simulink model "NHR9410Model96k_2020b"  (R2020b)
settings: Solver=ode45  StartTime=0.0  StopTime=1  FixedStep=0.001  MaxStep=20e-6  RelTol=1e-3
undefined symbols (not defined in the file): Ts
libraries: simulink x85, fl_lib x49, powerlib_meascontrol x27, simulink_extras x24, nesl_utility x13
(part 4 of 4)

== system NHR9410Model96k_2020b/NHR 9410 Safety Settings/Safety Ch-2/Trip signal generator (max) Sink Power/trip signal gen ==
  signal in : Inport
  Enable : EnablePort
  -1 : Constant  OutDataTypeStr=boolean
  -2 : Constant  OutDataTypeStr=boolean
  -3 : Constant  OutDataTypeStr=boolean
  -4 : Constant  Value=0  OutDataTypeStr=boolean
  -5 : Constant  Value=0  OutDataTypeStr=boolean
  -7 : Constant  Value=trip_t  OutDataTypeStr=boolean
  Add : Sum
  Compare To Constant : simulink/Logic and Bit Operations/Compare To Constant  relop=>  const=0  OutDataTypeStr=uint8
  Compare To Constant1 : simulink/Logic and Bit Operations/Compare To Constant  relop===  const=0  OutDataTypeStr=uint8
  D Latch1 : simulink_extras/Flip Flops/D Latch
      settings: SourceProductBaseCode=SL
  Data Type Conversion : DataTypeConversion  OutDataTypeStr=double
  Data Type Conversion1 : DataTypeConversion  OutDataTypeStr=double
  Gain : Gain  Gain=2
  Gain1 : Gain
  Logical Operator1 : Logic  AllPortsSameDT=off  OutDataTypeStr=boolean
  Multiport Switch : MultiPortSwitch  Inputs=2  DataPortForDefault=Additional data port
  On Delay : powerlib_meascontrol/Logic/On Delay  DelayType=On delay  delay=trip_t  ic=0  Ts=0
  Switch : Switch  Criteria=u2 > Threshold  Threshold=trip_thres
  Terminator1 : Terminator
  trip_out : Outport  VectorParamsAs1DForOutWhenUnconnected=off
  wires:
  Switch/1 -> On Delay/1, Logical Operator1/2
  On Delay/1 -> D Latch1/2
  D Latch1/1 -> Multiport Switch/2
  -4/1 -> Multiport Switch/4
  Multiport Switch/1 -> trip_out/1
  -2/1 -> Multiport Switch/3
  -3/1 -> Switch/1
  -5/1 -> Switch/3
  Logical Operator1/1 -> D Latch1/1
  D Latch1/2 -> Terminator1/1
  signal in/1 -> Switch/2
  -1/1 -> Logical Operator1/1
  -7/1 -> Compare To Constant1/1, Compare To Constant/1
  Gain1/1 -> Add/1
  Data Type Conversion/1 -> Gain1/1
  Add/1 -> Multiport Switch/1
  Gain/1 -> Add/2
  Data Type Conversion1/1 -> Gain/1
  Compare To Constant1/1 -> Data Type Conversion1/1
  Compare To Constant/1 -> Data Type Conversion/1

== system NHR9410Model96k_2020b/NHR 9410 Safety Settings/Safety Ch-2/Trip signal generator (max) Source Current/trip signal gen ==
  signal in : Inport
  Enable : EnablePort
  -1 : Constant  OutDataTypeStr=boolean
  -2 : Constant  OutDataTypeStr=boolean
  -3 : Constant  OutDataTypeStr=boolean
  -4 : Constant  Value=0  OutDataTypeStr=boolean
  -5 : Constant  Value=0  OutDataTypeStr=boolean
  -7 : Constant  Value=trip_t  OutDataTypeStr=boolean
  Add : Sum
  Compare To Constant : simulink/Logic and Bit Operations/Compare To Constant  relop=>  const=0  OutDataTypeStr=uint8
  Compare To Constant1 : simulink/Logic and Bit Operations/Compare To Constant  relop===  const=0  OutDataTypeStr=uint8
  D Latch1 : simulink_extras/Flip Flops/D Latch
      settings: SourceProductBaseCode=SL
  Data Type Conversion : DataTypeConversion  OutDataTypeStr=double
  Data Type Conversion1 : DataTypeConversion  OutDataTypeStr=double
  Gain : Gain  Gain=2
  Gain1 : Gain
  Logical Operator1 : Logic  AllPortsSameDT=off  OutDataTypeStr=boolean
  Multiport Switch : MultiPortSwitch  Inputs=2  DataPortForDefault=Additional data port
  On Delay : powerlib_meascontrol/Logic/On Delay  DelayType=On delay  delay=trip_t  ic=0  Ts=0
  Switch : Switch  Criteria=u2 > Threshold  Threshold=trip_thres
  Terminator1 : Terminator
  trip_out : Outport  VectorParamsAs1DForOutWhenUnconnected=off
  wires:
  Switch/1 -> On Delay/1, Logical Operator1/2
  On Delay/1 -> D Latch1/2
  D Latch1/1 -> Multiport Switch/2
  -4/1 -> Multiport Switch/4
  Multiport Switch/1 -> trip_out/1
  -2/1 -> Multiport Switch/3
  -3/1 -> Switch/1
  -5/1 -> Switch/3
  Logical Operator1/1 -> D Latch1/1
  D Latch1/2 -> Terminator1/1
  signal in/1 -> Switch/2
  -1/1 -> Logical Operator1/1
  -7/1 -> Compare To Constant1/1, Compare To Constant/1
  Gain1/1 -> Add/1
  Data Type Conversion/1 -> Gain1/1
  Add/1 -> Multiport Switch/1
  Gain/1 -> Add/2
  Data Type Conversion1/1 -> Gain/1
  Compare To Constant1/1 -> Data Type Conversion1/1
  Compare To Constant/1 -> Data Type Conversion/1

== system NHR9410Model96k_2020b/NHR 9410 Safety Settings/Safety Ch-2/Trip signal generator (max) Source Power/trip signal gen ==
  signal in : Inport
  Enable : EnablePort
  -1 : Constant  OutDataTypeStr=boolean
  -2 : Constant  OutDataTypeStr=boolean
  -3 : Constant  OutDataTypeStr=boolean
  -4 : Constant  Value=0  OutDataTypeStr=boolean
  -5 : Constant  Value=0  OutDataTypeStr=boolean
  -7 : Constant  Value=trip_t  OutDataTypeStr=boolean
  Add : Sum
  Compare To Constant : simulink/Logic and Bit Operations/Compare To Constant  relop=>  const=0  OutDataTypeStr=uint8
  Compare To Constant1 : simulink/Logic and Bit Operations/Compare To Constant  relop===  const=0  OutDataTypeStr=uint8
  D Latch1 : simulink_extras/Flip Flops/D Latch
      settings: SourceProductBaseCode=SL
  Data Type Conversion : DataTypeConversion  OutDataTypeStr=double
  Data Type Conversion1 : DataTypeConversion  OutDataTypeStr=double
  Gain : Gain  Gain=2
  Gain1 : Gain
  Logical Operator1 : Logic  AllPortsSameDT=off  OutDataTypeStr=boolean
  Multiport Switch : MultiPortSwitch  Inputs=2  DataPortForDefault=Additional data port
  On Delay : powerlib_meascontrol/Logic/On Delay  DelayType=On delay  delay=trip_t  ic=0  Ts=0
  Switch : Switch  Criteria=u2 > Threshold  Threshold=trip_thres
  Terminator1 : Terminator
  trip_out : Outport  VectorParamsAs1DForOutWhenUnconnected=off
  wires:
  -1/1 -> Logical Operator1/1
  signal in/1 -> Switch/2
  D Latch1/2 -> Terminator1/1
  Logical Operator1/1 -> D Latch1/1
  -5/1 -> Switch/3
  -3/1 -> Switch/1
  -2/1 -> Multiport Switch/3
  Multiport Switch/1 -> trip_out/1
  -4/1 -> Multiport Switch/4
  D Latch1/1 -> Multiport Switch/2
  On Delay/1 -> D Latch1/2
  Switch/1 -> Logical Operator1/2, On Delay/1
  -7/1 -> Compare To Constant1/1, Compare To Constant/1
  Gain1/1 -> Add/1
  Data Type Conversion/1 -> Gain1/1
  Add/1 -> Multiport Switch/1
  Gain/1 -> Add/2
  Data Type Conversion1/1 -> Gain/1
  Compare To Constant1/1 -> Data Type Conversion1/1
  Compare To Constant/1 -> Data Type Conversion/1

== system NHR9410Model96k_2020b/NHR 9410 Safety Settings/Safety Ch-2/Trip signal generator (max) Voltage/trip signal gen ==
  signal in : Inport
  Enable : EnablePort
  -1 : Constant  OutDataTypeStr=boolean
  -2 : Constant  OutDataTypeStr=boolean
  -3 : Constant  OutDataTypeStr=boolean
  -4 : Constant  Value=0  OutDataTypeStr=boolean
  -5 : Constant  Value=0  OutDataTypeStr=boolean
  -7 : Constant  Value=trip_t  OutDataTypeStr=boolean
  Add : Sum
  Compare To Constant : simulink/Logic and Bit Operations/Compare To Constant  relop=>  const=0  OutDataTypeStr=uint8
  Compare To Constant1 : simulink/Logic and Bit Operations/Compare To Constant  relop===  const=0  OutDataTypeStr=uint8
  D Latch1 : simulink_extras/Flip Flops/D Latch
      settings: SourceProductBaseCode=SL
  Data Type Conversion : DataTypeConversion  OutDataTypeStr=double
  Data Type Conversion1 : DataTypeConversion  OutDataTypeStr=double
  Gain : Gain  Gain=2
  Gain1 : Gain
  Logical Operator1 : Logic  AllPortsSameDT=off  OutDataTypeStr=boolean
  Multiport Switch : MultiPortSwitch  Inputs=2  DataPortForDefault=Additional data port
  On Delay : powerlib_meascontrol/Logic/On Delay  DelayType=On delay  delay=trip_t  ic=0  Ts=0
  Switch : Switch  Criteria=u2 > Threshold  Threshold=trip_thres
  Terminator1 : Terminator
  trip_out : Outport  VectorParamsAs1DForOutWhenUnconnected=off
  wires:
  -1/1 -> Logical Operator1/1
  signal in/1 -> Switch/2
  D Latch1/2 -> Terminator1/1
  Logical Operator1/1 -> D Latch1/1
  -5/1 -> Switch/3
  -3/1 -> Switch/1
  -2/1 -> Multiport Switch/3
  Multiport Switch/1 -> trip_out/1
  -4/1 -> Multiport Switch/4
  D Latch1/1 -> Multiport Switch/2
  On Delay/1 -> D Latch1/2
  Switch/1 -> Logical Operator1/2, On Delay/1
  -7/1 -> Compare To Constant1/1, Compare To Constant/1
  Gain1/1 -> Add/1
  Data Type Conversion/1 -> Gain1/1
  Add/1 -> Multiport Switch/1
  Gain/1 -> Add/2
  Data Type Conversion1/1 -> Gain/1
  Compare To Constant1/1 -> Data Type Conversion1/1
  Compare To Constant/1 -> Data Type Conversion/1

== system NHR9410Model96k_2020b/NHR 9410 Safety Settings/Safety Ch-2/Trip signal generator (min) Voltage/trip signal gen ==
  signal in : Inport
  Enable : EnablePort
  -1 : Constant  OutDataTypeStr=boolean
  -2 : Constant  OutDataTypeStr=boolean
  -3 : Constant  Value=0  OutDataTypeStr=boolean
  -4 : Constant  Value=0  OutDataTypeStr=boolean
  -5 : Constant  OutDataTypeStr=boolean
  -7 : Constant  Value=trip_t  OutDataTypeStr=boolean
  Add : Sum
  Compare To Constant : simulink/Logic and Bit Operations/Compare To Constant  relop=>  const=0  OutDataTypeStr=uint8
  Compare To Constant1 : simulink/Logic and Bit Operations/Compare To Constant  relop===  const=0  OutDataTypeStr=uint8
  D Latch1 : simulink_extras/Flip Flops/D Latch
      settings: SourceProductBaseCode=SL
  Data Type Conversion : DataTypeConversion  OutDataTypeStr=double
  Data Type Conversion1 : DataTypeConversion  OutDataTypeStr=double
  Gain : Gain  Gain=2
  Gain1 : Gain
  Logical Operator1 : Logic  AllPortsSameDT=off  OutDataTypeStr=boolean
  Multiport Switch : MultiPortSwitch  Inputs=2  DataPortForDefault=Additional data port
  On Delay : powerlib_meascontrol/Logic/On Delay  DelayType=On delay  delay=trip_t  ic=0  Ts=0
  Switch : Switch  Criteria=u2 > Threshold  Threshold=trip_thres
  Terminator1 : Terminator
  trip_out : Outport  VectorParamsAs1DForOutWhenUnconnected=off
  wires:
  Switch/1 -> On Delay/1, Logical Operator1/2
  On Delay/1 -> D Latch1/2
  D Latch1/1 -> Multiport Switch/2
  -4/1 -> Multiport Switch/4
  Multiport Switch/1 -> trip_out/1
  -2/1 -> Multiport Switch/3
  -3/1 -> Switch/1
  -5/1 -> Switch/3
  Logical Operator1/1 -> D Latch1/1
  D Latch1/2 -> Terminator1/1
  signal in/1 -> Switch/2
  -1/1 -> Logical Operator1/1
  -7/1 -> Compare To Constant1/1, Compare To Constant/1
  Gain1/1 -> Add/1
  Data Type Conversion/1 -> Gain1/1
  Add/1 -> Multiport Switch/1
  Gain/1 -> Add/2
  Data Type Conversion1/1 -> Gain/1
  Compare To Constant1/1 -> Data Type Conversion1/1
  Compare To Constant/1 -> Data Type Conversion/1

== system NHR9410Model96k_2020b/NHR 9410 Safety Settings/Safety Ch-2/Trip signal generator (peak) Current/trip signal gen ==
  signal in : Inport
  Enable : EnablePort
  -2 : Constant  OutDataTypeStr=boolean
  -4 : Constant  Value=0  OutDataTypeStr=boolean
  D Latch1 : simulink_extras/Flip Flops/D Latch
      settings: SourceProductBaseCode=SL
  Data Type Conversion : DataTypeConversion  OutDataTypeStr=boolean
  Switch1 : Switch  Criteria=u2 > Threshold  Threshold=trip_thres
  Terminator1 : Terminator
  trip_out : Outport  VectorParamsAs1DForOutWhenUnconnected=off
  wires:
  -4/1 -> Switch1/3
  Switch1/1 -> D Latch1/2, Data Type Conversion/1
  D Latch1/1 -> trip_out/1
  D Latch1/2 -> Terminator1/1
  -2/1 -> Switch1/1
  Data Type Conversion/1 -> D Latch1/1
  signal in/1 -> Switch1/2

== system NHR9410Model96k_2020b/NHR 9410 Safety Settings/Safety Ch-2/Trip signal generator (peak) Voltage/trip signal gen ==
  signal in : Inport
  Enable : EnablePort
  -2 : Constant  OutDataTypeStr=boolean
  -4 : Constant  Value=0  OutDataTypeStr=boolean
  D Latch1 : simulink_extras/Flip Flops/D Latch
      settings: SourceProductBaseCode=SL
  Data Type Conversion : DataTypeConversion  OutDataTypeStr=boolean
  Switch1 : Switch  Criteria=u2 > Threshold  Threshold=trip_thres
  Terminator1 : Terminator
  trip_out : Outport  VectorParamsAs1DForOutWhenUnconnected=off
  wires:
  -4/1 -> Switch1/3
  Switch1/1 -> D Latch1/2, Data Type Conversion/1
  D Latch1/1 -> trip_out/1
  D Latch1/2 -> Terminator1/1
  -2/1 -> Switch1/1
  Data Type Conversion/1 -> D Latch1/1
  signal in/1 -> Switch1/2

== system NHR9410Model96k_2020b/NHR 9410 Safety Settings/Safety Ch-3/Trip signal generator (max) Sink Current/trip signal gen ==
  signal in : Inport
  Enable : EnablePort
  -1 : Constant  OutDataTypeStr=boolean
  -2 : Constant  OutDataTypeStr=boolean
  -3 : Constant  OutDataTypeStr=boolean
  -4 : Constant  Value=0  OutDataTypeStr=boolean
  -5 : Constant  Value=0  OutDataTypeStr=boolean
  -7 : Constant  Value=trip_t  OutDataTypeStr=boolean
  Add : Sum
  Compare To Constant : simulink/Logic and Bit Operations/Compare To Constant  relop=>  const=0  OutDataTypeStr=uint8
  Compare To Constant1 : simulink/Logic and Bit Operations/Compare To Constant  relop===  const=0  OutDataTypeStr=uint8
  D Latch1 : simulink_extras/Flip Flops/D Latch
      settings: SourceProductBaseCode=SL
  Data Type Conversion : DataTypeConversion  OutDataTypeStr=double
  Data Type Conversion1 : DataTypeConversion  OutDataTypeStr=double
  Gain : Gain  Gain=2
  Gain1 : Gain
  Logical Operator1 : Logic  AllPortsSameDT=off  OutDataTypeStr=boolean
  Multiport Switch : MultiPortSwitch  Inputs=2  DataPortForDefault=Additional data port
  On Delay : powerlib_meascontrol/Logic/On Delay  DelayType=On delay  delay=trip_t  ic=0  Ts=0
  Switch : Switch  Criteria=u2 > Threshold  Threshold=trip_thres
  Terminator1 : Terminator
  trip_out : Outport  VectorParamsAs1DForOutWhenUnconnected=off
  wires:
  Switch/1 -> On Delay/1, Logical Operator1/2
  On Delay/1 -> D Latch1/2
  D Latch1/1 -> Multiport Switch/2
  -4/1 -> Multiport Switch/4
  Multiport Switch/1 -> trip_out/1
  -2/1 -> Multiport Switch/3
  -3/1 -> Switch/1
  -5/1 -> Switch/3
  Logical Operator1/1 -> D Latch1/1
  D Latch1/2 -> Terminator1/1
  signal in/1 -> Switch/2
  -1/1 -> Logical Operator1/1
  -7/1 -> Compare To Constant1/1, Compare To Constant/1
  Gain1/1 -> Add/1
  Data Type Conversion/1 -> Gain1/1
  Add/1 -> Multiport Switch/1
  Gain/1 -> Add/2
  Data Type Conversion1/1 -> Gain/1
  Compare To Constant1/1 -> Data Type Conversion1/1
  Compare To Constant/1 -> Data Type Conversion/1

== system NHR9410Model96k_2020b/NHR 9410 Safety Settings/Safety Ch-3/Trip signal generator (max) Sink Power/trip signal gen ==
  signal in : Inport
  Enable : EnablePort
  -1 : Constant  OutDataTypeStr=boolean
  -2 : Constant  OutDataTypeStr=boolean
  -3 : Constant  OutDataTypeStr=boolean
  -4 : Constant  Value=0  OutDataTypeStr=boolean
  -5 : Constant  Value=0  OutDataTypeStr=boolean
  -7 : Constant  Value=trip_t  OutDataTypeStr=boolean
  Add : Sum
  Compare To Constant : simulink/Logic and Bit Operations/Compare To Constant  relop=>  const=0  OutDataTypeStr=uint8
  Compare To Constant1 : simulink/Logic and Bit Operations/Compare To Constant  relop===  const=0  OutDataTypeStr=uint8
  D Latch1 : simulink_extras/Flip Flops/D Latch
      settings: SourceProductBaseCode=SL
  Data Type Conversion : DataTypeConversion  OutDataTypeStr=double
  Data Type Conversion1 : DataTypeConversion  OutDataTypeStr=double
  Gain : Gain  Gain=2
  Gain1 : Gain
  Logical Operator1 : Logic  AllPortsSameDT=off  OutDataTypeStr=boolean
  Multiport Switch : MultiPortSwitch  Inputs=2  DataPortForDefault=Additional data port
  On Delay : powerlib_meascontrol/Logic/On Delay  DelayType=On delay  delay=trip_t  ic=0  Ts=0
  Switch : Switch  Criteria=u2 > Threshold  Threshold=trip_thres
  Terminator1 : Terminator
  trip_out : Outport  VectorParamsAs1DForOutWhenUnconnected=off
  wires:
  -1/1 -> Logical Operator1/1
  signal in/1 -> Switch/2
  D Latch1/2 -> Terminator1/1
  Logical Operator1/1 -> D Latch1/1
  -5/1 -> Switch/3
  -3/1 -> Switch/1
  -2/1 -> Multiport Switch/3
  Multiport Switch/1 -> trip_out/1
  -4/1 -> Multiport Switch/4
  D Latch1/1 -> Multiport Switch/2
  On Delay/1 -> D Latch1/2
  Switch/1 -> Logical Operator1/2, On Delay/1
  -7/1 -> Compare To Constant1/1, Compare To Constant/1
  Gain1/1 -> Add/1
  Data Type Conversion/1 -> Gain1/1
  Add/1 -> Multiport Switch/1
  Gain/1 -> Add/2
  Data Type Conversion1/1 -> Gain/1
  Compare To Constant1/1 -> Data Type Conversion1/1
  Compare To Constant/1 -> Data Type Conversion/1

== system NHR9410Model96k_2020b/NHR 9410 Safety Settings/Safety Ch-3/Trip signal generator (max) Source Current/trip signal gen ==
  signal in : Inport
  Enable : EnablePort
  -1 : Constant  OutDataTypeStr=boolean
  -2 : Constant  OutDataTypeStr=boolean
  -3 : Constant  OutDataTypeStr=boolean
  -4 : Constant  Value=0  OutDataTypeStr=boolean
  -5 : Constant  Value=0  OutDataTypeStr=boolean
  -7 : Constant  Value=trip_t  OutDataTypeStr=boolean
  Add : Sum
  Compare To Constant : simulink/Logic and Bit Operations/Compare To Constant  relop=>  const=0  OutDataTypeStr=uint8
  Compare To Constant1 : simulink/Logic and Bit Operations/Compare To Constant  relop===  const=0  OutDataTypeStr=uint8
  D Latch1 : simulink_extras/Flip Flops/D Latch
      settings: SourceProductBaseCode=SL
  Data Type Conversion : DataTypeConversion  OutDataTypeStr=double
  Data Type Conversion1 : DataTypeConversion  OutDataTypeStr=double
  Gain : Gain  Gain=2
  Gain1 : Gain
  Logical Operator1 : Logic  AllPortsSameDT=off  OutDataTypeStr=boolean
  Multiport Switch : MultiPortSwitch  Inputs=2  DataPortForDefault=Additional data port
  On Delay : powerlib_meascontrol/Logic/On Delay  DelayType=On delay  delay=trip_t  ic=0  Ts=0
  Switch : Switch  Criteria=u2 > Threshold  Threshold=trip_thres
  Terminator1 : Terminator
  trip_out : Outport  VectorParamsAs1DForOutWhenUnconnected=off
  wires:
  -1/1 -> Logical Operator1/1
  signal in/1 -> Switch/2
  D Latch1/2 -> Terminator1/1
  Logical Operator1/1 -> D Latch1/1
  -5/1 -> Switch/3
  -3/1 -> Switch/1
  -2/1 -> Multiport Switch/3
  Multiport Switch/1 -> trip_out/1
  -4/1 -> Multiport Switch/4
  D Latch1/1 -> Multiport Switch/2
  On Delay/1 -> D Latch1/2
  Switch/1 -> Logical Operator1/2, On Delay/1
  -7/1 -> Compare To Constant1/1, Compare To Constant/1
  Gain1/1 -> Add/1
  Data Type Conversion/1 -> Gain1/1
  Add/1 -> Multiport Switch/1
  Gain/1 -> Add/2
  Data Type Conversion1/1 -> Gain/1
  Compare To Constant1/1 -> Data Type Conversion1/1
  Compare To Constant/1 -> Data Type Conversion/1

== system NHR9410Model96k_2020b/NHR 9410 Safety Settings/Safety Ch-3/Trip signal generator (max) Source Power/trip signal gen ==
  signal in : Inport
  Enable : EnablePort
  -1 : Constant  OutDataTypeStr=boolean
  -2 : Constant  OutDataTypeStr=boolean
  -3 : Constant  OutDataTypeStr=boolean
  -4 : Constant  Value=0  OutDataTypeStr=boolean
  -5 : Constant  Value=0  OutDataTypeStr=boolean
  -7 : Constant  Value=trip_t  OutDataTypeStr=boolean
  Add : Sum
  Compare To Constant : simulink/Logic and Bit Operations/Compare To Constant  relop=>  const=0  OutDataTypeStr=uint8
  Compare To Constant1 : simulink/Logic and Bit Operations/Compare To Constant  relop===  const=0  OutDataTypeStr=uint8
  D Latch1 : simulink_extras/Flip Flops/D Latch
      settings: SourceProductBaseCode=SL
  Data Type Conversion : DataTypeConversion  OutDataTypeStr=double
  Data Type Conversion1 : DataTypeConversion  OutDataTypeStr=double
  Gain : Gain  Gain=2
  Gain1 : Gain
  Logical Operator1 : Logic  AllPortsSameDT=off  OutDataTypeStr=boolean
  Multiport Switch : MultiPortSwitch  Inputs=2  DataPortForDefault=Additional data port
  On Delay : powerlib_meascontrol/Logic/On Delay  DelayType=On delay  delay=trip_t  ic=0  Ts=0
  Switch : Switch  Criteria=u2 > Threshold  Threshold=trip_thres
  Terminator1 : Terminator
  trip_out : Outport  VectorParamsAs1DForOutWhenUnconnected=off
  wires:
  Switch/1 -> On Delay/1, Logical Operator1/2
  On Delay/1 -> D Latch1/2
  D Latch1/1 -> Multiport Switch/2
  -4/1 -> Multiport Switch/4
  Multiport Switch/1 -> trip_out/1
  -2/1 -> Multiport Switch/3
  -3/1 -> Switch/1
  -5/1 -> Switch/3
  Logical Operator1/1 -> D Latch1/1
  D Latch1/2 -> Terminator1/1
  signal in/1 -> Switch/2
  -1/1 -> Logical Operator1/1
  -7/1 -> Compare To Constant1/1, Compare To Constant/1
  Gain1/1 -> Add/1
  Data Type Conversion/1 -> Gain1/1
  Add/1 -> Multiport Switch/1
  Gain/1 -> Add/2
  Data Type Conversion1/1 -> Gain/1
  Compare To Constant1/1 -> Data Type Conversion1/1
  Compare To Constant/1 -> Data Type Conversion/1

== system NHR9410Model96k_2020b/NHR 9410 Safety Settings/Safety Ch-3/Trip signal generator (max) Voltage/trip signal gen ==
  signal in : Inport
  Enable : EnablePort
  -1 : Constant  OutDataTypeStr=boolean
  -2 : Constant  OutDataTypeStr=boolean
  -3 : Constant  OutDataTypeStr=boolean
  -4 : Constant  Value=0  OutDataTypeStr=boolean
  -5 : Constant  Value=0  OutDataTypeStr=boolean
  -7 : Constant  Value=trip_t  OutDataTypeStr=boolean
  Add : Sum
  Compare To Constant : simulink/Logic and Bit Operations/Compare To Constant  relop=>  const=0  OutDataTypeStr=uint8
  Compare To Constant1 : simulink/Logic and Bit Operations/Compare To Constant  relop===  const=0  OutDataTypeStr=uint8
  D Latch1 : simulink_extras/Flip Flops/D Latch
      settings: SourceProductBaseCode=SL
  Data Type Conversion : DataTypeConversion  OutDataTypeStr=double
  Data Type Conversion1 : DataTypeConversion  OutDataTypeStr=double
  Gain : Gain  Gain=2
  Gain1 : Gain
  Logical Operator1 : Logic  AllPortsSameDT=off  OutDataTypeStr=boolean
  Multiport Switch : MultiPortSwitch  Inputs=2  DataPortForDefault=Additional data port
  On Delay : powerlib_meascontrol/Logic/On Delay  DelayType=On delay  delay=trip_t  ic=0  Ts=0
  Switch : Switch  Criteria=u2 > Threshold  Threshold=trip_thres
  Terminator1 : Terminator
  trip_out : Outport  VectorParamsAs1DForOutWhenUnconnected=off
  wires:
  Switch/1 -> On Delay/1, Logical Operator1/2
  On Delay/1 -> D Latch1/2
  D Latch1/1 -> Multiport Switch/2
  -4/1 -> Multiport Switch/4
  Multiport Switch/1 -> trip_out/1
  -2/1 -> Multiport Switch/3
  -3/1 -> Switch/1
  -5/1 -> Switch/3
  Logical Operator1/1 -> D Latch1/1
  D Latch1/2 -> Terminator1/1
  signal in/1 -> Switch/2
  -1/1 -> Logical Operator1/1
  -7/1 -> Compare To Constant1/1, Compare To Constant/1
  Gain1/1 -> Add/1
  Data Type Conversion/1 -> Gain1/1
  Add/1 -> Multiport Switch/1
  Gain/1 -> Add/2
  Data Type Conversion1/1 -> Gain/1
  Compare To Constant1/1 -> Data Type Conversion1/1
  Compare To Constant/1 -> Data Type Conversion/1

== system NHR9410Model96k_2020b/NHR 9410 Safety Settings/Safety Ch-3/Trip signal generator (min) Voltage/trip signal gen ==
  signal in : Inport
  Enable : EnablePort
  -1 : Constant  OutDataTypeStr=boolean
  -2 : Constant  OutDataTypeStr=boolean
  -3 : Constant  Value=0  OutDataTypeStr=boolean
  -4 : Constant  Value=0  OutDataTypeStr=boolean
  -5 : Constant  OutDataTypeStr=boolean
  -7 : Constant  Value=trip_t  OutDataTypeStr=boolean
  Add : Sum
  Compare To Constant : simulink/Logic and Bit Operations/Compare To Constant  relop=>  const=0  OutDataTypeStr=uint8
  Compare To Constant1 : simulink/Logic and Bit Operations/Compare To Constant  relop===  const=0  OutDataTypeStr=uint8
  D Latch1 : simulink_extras/Flip Flops/D Latch
      settings: SourceProductBaseCode=SL
  Data Type Conversion : DataTypeConversion  OutDataTypeStr=double
  Data Type Conversion1 : DataTypeConversion  OutDataTypeStr=double
  Gain : Gain  Gain=2
  Gain1 : Gain
  Logical Operator1 : Logic  AllPortsSameDT=off  OutDataTypeStr=boolean
  Multiport Switch : MultiPortSwitch  Inputs=2  DataPortForDefault=Additional data port
  On Delay : powerlib_meascontrol/Logic/On Delay  DelayType=On delay  delay=trip_t  ic=0  Ts=0
  Switch : Switch  Criteria=u2 > Threshold  Threshold=trip_thres
  Terminator1 : Terminator
  trip_out : Outport  VectorParamsAs1DForOutWhenUnconnected=off
  wires:
  -1/1 -> Logical Operator1/1
  signal in/1 -> Switch/2
  D Latch1/2 -> Terminator1/1
  Logical Operator1/1 -> D Latch1/1
  -5/1 -> Switch/3
  -3/1 -> Switch/1
  -2/1 -> Multiport Switch/3
  Multiport Switch/1 -> trip_out/1
  -4/1 -> Multiport Switch/4
  D Latch1/1 -> Multiport Switch/2
  On Delay/1 -> D Latch1/2
  Switch/1 -> Logical Operator1/2, On Delay/1
  -7/1 -> Compare To Constant1/1, Compare To Constant/1
  Gain1/1 -> Add/1
  Data Type Conversion/1 -> Gain1/1
  Add/1 -> Multiport Switch/1
  Gain/1 -> Add/2
  Data Type Conversion1/1 -> Gain/1
  Compare To Constant1/1 -> Data Type Conversion1/1
  Compare To Constant/1 -> Data Type Conversion/1

== system NHR9410Model96k_2020b/NHR 9410 Safety Settings/Safety Ch-3/Trip signal generator (peak) Current/trip signal gen ==
  signal in : Inport
  Enable : EnablePort
  -2 : Constant  OutDataTypeStr=boolean
  -4 : Constant  Value=0  OutDataTypeStr=boolean
  D Latch1 : simulink_extras/Flip Flops/D Latch
      settings: SourceProductBaseCode=SL
  Data Type Conversion : DataTypeConversion  OutDataTypeStr=boolean
  Switch1 : Switch  Criteria=u2 > Threshold  Threshold=trip_thres
  Terminator1 : Terminator
  trip_out : Outport  VectorParamsAs1DForOutWhenUnconnected=off
  wires:
  -4/1 -> Switch1/3
  Switch1/1 -> D Latch1/2, Data Type Conversion/1
  D Latch1/1 -> trip_out/1
  D Latch1/2 -> Terminator1/1
  -2/1 -> Switch1/1
  Data Type Conversion/1 -> D Latch1/1
  signal in/1 -> Switch1/2

== system NHR9410Model96k_2020b/NHR 9410 Safety Settings/Safety Ch-3/Trip signal generator (peak) Voltage/trip signal gen ==
  signal in : Inport
  Enable : EnablePort
  -2 : Constant  OutDataTypeStr=boolean
  -4 : Constant  Value=0  OutDataTypeStr=boolean
  D Latch1 : simulink_extras/Flip Flops/D Latch
      settings: SourceProductBaseCode=SL
  Data Type Conversion : DataTypeConversion  OutDataTypeStr=boolean
  Switch1 : Switch  Criteria=u2 > Threshold  Threshold=trip_thres
  Terminator1 : Terminator
  trip_out : Outport  VectorParamsAs1DForOutWhenUnconnected=off
  wires:
  -4/1 -> Switch1/3
  Switch1/1 -> D Latch1/2, Data Type Conversion/1
  D Latch1/1 -> trip_out/1
  D Latch1/2 -> Terminator1/1
  -2/1 -> Switch1/1
  Data Type Conversion/1 -> D Latch1/1
  signal in/1 -> Switch1/2

== matlab function NHR9410Model96k_2020b/NHR 9410/Chanel-3/Chanel-3 Control/All DC (mode-4) control1/MATLAB Function ==
  data: p input; v input; y output; i input; x input
function y = fcn(p,v,i,x)
tol=1e-3;
gain=1e-4;
Ts=1e-3;
if p<=(-tol)
    y=x-(gain/Ts);
elseif i<=(-tol)
    y=x-(gain/Ts);
elseif v<=(-tol)
    y=x-(gain/Ts);
elseif v>tol;
    y=x+(gain/Ts);
else
    y=0;
end

== matlab function NHR9410Model96k_2020b/NHR 9410/Chanel-1/Chanel-1 Control/All AC control/MATLAB Function ==
  data: p input; v input; y output; i input; x input
function y = fcn(p,v,i,x)
tol=1e-3;
gain=1e-4;
Ts=1e-3;
if p<=(-tol)
    y=x-(gain/Ts);
elseif i<=(-tol)
    y=x-(gain/Ts);
elseif v<=(-tol)
    y=x-(gain/Ts);
elseif v>tol;
    y=x+(gain/Ts);
else
    y=0;
end

== matlab function NHR9410Model96k_2020b/NHR 9410/Chanel-3/Chanel-3 Control/Three AC (mode-3) control1/MATLAB Function ==
  data: p input; v input; y output; i input; x input
function y = fcn(p,v,i,x)
tol=1e-3;
gain=1e-4;
Ts=1e-3;
if p<=(-tol)
    y=x-(gain/Ts);
elseif i<=(-tol)
    y=x-(gain/Ts);
elseif v<=(-tol)
    y=x-(gain/Ts);
elseif v>tol;
    y=x+(gain/Ts);
else
    y=0;
end

== matlab function NHR9410Model96k_2020b/NHR 9410/Chanel-1/Chanel-1 Control/All AC control/MATLAB Function2 ==
  data: t input; y output; Vrms input; F input; theta1 input
function y = fcn(t,Vrms,F,theta1)
y = sqrt(2)*Vrms*sin(2*pi*F*t + theta1*pi/180);

== matlab function NHR9410Model96k_2020b/NHR 9410/Chanel-1/Chanel-1 Control/All DC control/MATLAB Function ==
  data: p input; v input; y output; i input; x input
function y = fcn(p,v,i,x)
tol=1e-3;
gain=1e-4;
Ts=1e-3;
if p<=(-tol)
    y=x-(gain/Ts);
elseif i<=(-tol)
    y=x-(gain/Ts);
elseif v<=(-tol)
    y=x-(gain/Ts);
elseif v>tol;
    y=x+(gain/Ts);
else
    y=0;
end

== matlab function NHR9410Model96k_2020b/NHR 9410/Chanel-3/Chanel-3 Control/Three AC (mode-3) control1/MATLAB Function2 ==
  data: t input; y output; Vrms input; F input; theta1 input
function y = fcn(t,Vrms,F,theta1)
y = sqrt(2)*Vrms*sin(2*pi*F*t + theta1*pi/180);

== matlab function NHR9410Model96k_2020b/NHR 9410/Chanel-2/Chanel-2 Control1/All DC control/MATLAB Function ==
  data: p input; v input; y output; i input; x input
function y = fcn(p,v,i,x)
tol=1e-3;
gain=1e-4;
Ts=1e-3;
if p<=(-tol)
    y=x-(gain/Ts);
elseif i<=(-tol)
    y=x-(gain/Ts);
elseif v<=(-tol)
    y=x-(gain/Ts);
elseif v>tol;
    y=x+(gain/Ts);
else
    y=0;
end

== matlab function NHR9410Model96k_2020b/NHR 9410/Chanel-2/Chanel-2 Control1/All AC control/MATLAB Function ==
  data: p input; v input; y output; i input; x input
function y = fcn(p,v,i,x)
tol=1e-3;
gain=1e-4;
Ts=1e-3;
if p<=(-tol)
    y=x-(gain/Ts);
elseif i<=(-tol)
    y=x-(gain/Ts);
elseif v<=(-tol)
    y=x-(gain/Ts);
elseif v>tol;
    y=x+(gain/Ts);
else
    y=0;
end

== matlab function NHR9410Model96k_2020b/NHR 9410/Chanel-2/Chanel-2 Control1/All AC control/MATLAB Function2 ==
  data: t input; y output; Vrms input; F input; theta1 input
function y = fcn(t,Vrms,F,theta1)
y = sqrt(2)*Vrms*sin(2*pi*F*t + theta1*pi/180);
